simulink model "BD_PAR_AUTO_base_model"  (Simulink 10.3)
settings: Solver=ode1  StartTime=0.0  StopTime=max(cyc_mph(:,1))  FixedStep=1  MaxStep=1  RelTol=1e-3  AbsTol=1e-3
undefined symbols (not defined in the file): acc_dcdc_eff, acc_elec_eff, acc_elec_pwr, acc_mech_eff, acc_mech_pwr, acc_mech_trq, air_cp, amb_tmp, cs_charge_deplete_bool, cs_charge_trq, cs_electric_decel_spd, cs_electric_launch_spd_hi, cs_electric_launch_spd_lo, cs_hi_soc, cs_lo_soc, cs_min_trq_frac, cs_off_trq_frac, cyc_avg_time, cyc_cargo_mass, cyc_elevation_init, cyc_filter_bool, cyc_grade, cyc_mph, enable_sim_stop_distance, enable_sim_stop_max_spd, enable_sim_stop_speed, enable_sim_stop_time, enable_stop, enable_stop_fc, ess_cap_scale, ess_coulombic_eff, ess_init_soc, ess_max_ah_cap, ess_max_volts, ess_min_volts, ess_mod_airflow, ess_mod_cp, ess_mod_init_tmp, ess_module_mass, ess_module_num, ess_on, ess_r_chg, ess_r_dis, ess_res_scale_coef, ess_res_scale_fun, ess_set_tmp, ess_soc, ess_th_calc, ess_th_res_off, ess_th_res_on, ess_tmp, ess_voc, ex_calc, ex_cat_co_frac, ex_cat_ext_cp, ex_cat_ext_emisv, ex_cat_ext_init_tmp, ex_cat_ext_mass, ex_cat_ext_sarea, ex_cat_hc_frac ... (+168)
(part 7 of 15)

== system BD_PAR_AUTO_base_model/energy storage <ess>/ess config/energy storage <ess>/pack Voc, Rint ==
  SOC (prev) : Inport
  req'd battery power (W) : Inport  Port=2
  mod tmp   (C) : Inport  Port=3
  #bty : Constant  Value=ess_module_num
  Product : Product  InputSameDT=on  RndMeth=Zero  SaturateOnIntegerOverflow=on  OutDataTypeStr=Inherit: Same as first input
  Rchg (ohms) : Subsystem  mask(2-D Table Lookup){xindex=ess_tmp, yindex=ess_soc, table=ess_r_chg}
      mask prompts: xindex "X Index"; yindex "Y Index"
      mask help:
      | Two Dimensional Table Lookup
      | The first input corresponds to X Index and the second input corresponds to the Y Index
      mask init:
      | sftab2chk(xindex,yindex,table);
      mask Help: This block returns a linearly interpolated intersection from the table using the X index (which corresponds to the rows of the table) and the Y index (which corresponds to the columns of the table).  Extrapolation is used.
      mask Display: plot(-10,-10,110,110,[90,50,10],[90,40,30],[90,50,10],[50,26,20],[90,50,10],[22,13,10])
  Rdis (ohms) : Subsystem  mask(2-D Table Lookup){xindex=ess_tmp, yindex=ess_soc, table=ess_r_dis}
      mask prompts: xindex "X Index"; yindex "Y Index"
      mask help:
      | Two Dimensional Table Lookup
      | The first input corresponds to X Index and the second input corresponds to the Y Index
      mask init:
      | sftab2chk(xindex,yindex,table);
      mask Help: This block returns a linearly interpolated intersection from the table using the X index (which corresponds to the rows of the table) and the Y index (which corresponds to the columns of the table).  Extrapolation is used.
      mask Display: plot(-10,-10,110,110,[90,50,10],[90,40,30],[90,50,10],[50,26,20],[90,50,10],[22,13,10])
  Switch : Switch
  VOC (V) : Subsystem  mask(2-D Table Lookup){xindex=ess_tmp, yindex=ess_soc, table=ess_voc}
      mask prompts: xindex "X Index"; yindex "Y Index"
      mask help:
      | Two Dimensional Table Lookup
      | The first input corresponds to X Index and the second input corresponds to the Y Index
      mask init:
      | sftab2chk(xindex,yindex,table);
      mask Help: This block returns a linearly interpolated intersection from the table using the X index (which corresponds to the rows of the table) and the Y index (which corresponds to the columns of the table).  Extrapolation is used.
      mask Display: plot(-10,-10,110,110,[90,50,10],[90,40,30],[90,50,10],[50,26,20],[90,50,10],[22,13,10])
  resistance scale fun : Gain  Gain=ess_res_scale_fun(ess_res_scale_coef,ess_module_num,ess_cap_scale)  SaturateOnIntegerOverflow=on  OutDataTypeStr=Inherit: Same as input  ParamDataTypeStr=Inherit: Same as input
  resistance scale fun1 : Gain  Gain=ess_res_scale_fun(ess_res_scale_coef,ess_module_num,ess_cap_scale)  SaturateOnIntegerOverflow=on  OutDataTypeStr=Inherit: Same as input  ParamDataTypeStr=Inherit: Same as input
  pack open- circuit voltage : Outport  InitialOutput=0
  pack resistance : Outport  Port=2  InitialOutput=0
  wires:
  resistance scale fun1/1 -> Switch/3
  Rchg (ohms)/1(table out) -> resistance scale fun1/1
  resistance scale fun/1 -> Switch/1
  Rdis (ohms)/1(table out) -> resistance scale fun/1
  Switch/1 -> pack resistance/1
  #bty/1 -> Product/2
  Product/1 -> pack open- circuit voltage/1
  VOC (V)/1(table out) -> Product/1
  req'd battery power (W)/1 -> Switch/2
  SOC (prev)/1 -> VOC (V)/2(y0), Rdis (ohms)/2(y0), Rchg (ohms)/2(y0)
  mod tmp   (C)/1 -> VOC (V)/1(x0), Rdis (ohms)/1(x0), Rchg (ohms)/1(x0)

== system BD_PAR_AUTO_base_model/energy storage <ess>/ess config/energy storage <ess>/stop sim ==
  SOC : Inport
  Enable : EnablePort
  Const : Constant  Value=.001
  Relational Operator : RelationalOperator  Operator=<  RndMeth=Nearest  InputSameDT=on
  Stop Simulation : Stop
  wires:
  Const/1 -> Relational Operator/2
  SOC/1 -> Relational Operator/1
  Relational Operator/1 -> Stop Simulation/1

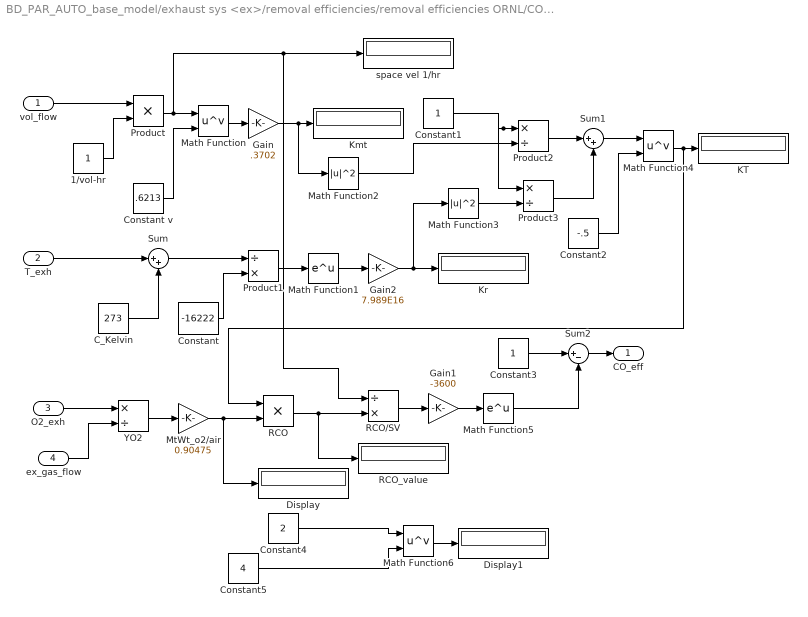
== system BD_PAR_AUTO_base_model/exhaust sys <ex>/removal efficiencies/removal efficiencies ORNL/CO-Conversion ==
  vol_flow : Inport
  T_exh : Inport  Port=2
  O2_exh : Inport  Port=3
  ex_gas_flow : Inport  Port=4
  1/vol-hr : Constant
  C_Kelvin : Constant  Value=273
  Constant : Constant  Value=-16222
  Constant v : Constant  Value=.6213
  Constant1 : Constant
  Constant2 : Constant  Value=-.5
  Constant3 : Constant
  Constant4 : Constant  Value=2
  Constant5 : Constant  Value=4
  Display : Display
  Display1 : Display
  Gain : Gain  Gain=.3702  SaturateOnIntegerOverflow=on
  Gain1 : Gain  Gain=-3600  SaturateOnIntegerOverflow=on
  Gain2 : Gain  Gain=7.989E16  SaturateOnIntegerOverflow=on
  KT : Display
      settings: Format=short_e
  Kmt : Display
      settings: Format=short_e
  Kr : Display
  Math Function : Math  Operator=pow
  Math Function1 : Math
  Math Function2 : Math  Operator=magnitude^2
  Math Function3 : Math  Operator=magnitude^2
  Math Function4 : Math  Operator=pow
  Math Function5 : Math
  Math Function6 : Math  Operator=pow
  MtWt_o2/air : Gain  Gain=0.90475  SaturateOnIntegerOverflow=on
  Product : Product  SaturateOnIntegerOverflow=on
  Product1 : Product  Inputs=/*  SaturateOnIntegerOverflow=on
  Product2 : Product  Inputs=*/  SaturateOnIntegerOverflow=on
  Product3 : Product  Inputs=*/  SaturateOnIntegerOverflow=on
  RCO : Product  SaturateOnIntegerOverflow=on
  RCO/SV : Product  Inputs=/*  SaturateOnIntegerOverflow=on
  RCO_value : Display
  Sum : Sum  Inputs=|++  SaturateOnIntegerOverflow=on
  Sum1 : Sum  Inputs=|++  SaturateOnIntegerOverflow=on
  Sum2 : Sum  Inputs=|+-  SaturateOnIntegerOverflow=on
  YO2 : Product  Inputs=*/  SaturateOnIntegerOverflow=on
  space vel 1/hr : Display
      settings: Format=short_e
  CO_eff : Outport
  wires:
  Math Function6/1 -> Display1/1
  Constant5/1 -> Math Function6/2
  Constant4/1 -> Math Function6/1
  MtWt_o2/air/1 -> Display/1, RCO/2
  YO2/1 -> MtWt_o2/air/1
  RCO/1 -> RCO_value/1, RCO/SV/2
  Sum2/1 -> CO_eff/1
  Math Function5/1 -> Sum2/2
  Constant3/1 -> Sum2/1
  Gain1/1 -> Math Function5/1
  RCO/SV/1 -> Gain1/1
  Math Function4/1 -> RCO/1, KT/1
  ex_gas_flow/1 -> YO2/2
  O2_exh/1 -> YO2/1
  T_exh/1 -> Sum/1
  vol_flow/1 -> Product/1
  Product1/1 -> Math Function1/1
  Constant2/1 -> Math Function4/2
  Sum1/1 -> Math Function4/1
  Product3/1 -> Sum1/2
  Product2/1 -> Sum1/1
  Math Function3/1 -> Product3/2
  Math Function2/1 -> Product2/2
  Constant1/1 -> Product2/1, Product3/1
  Gain2/1 -> Math Function3/1, Kr/1
  Gain/1 -> Math Function2/1, Kmt/1
  Math Function1/1 -> Gain2/1
  Sum/1 -> Product1/1
  Constant/1 -> Product1/2
  C_Kelvin/1 -> Sum/2
  Product/1 -> RCO/SV/1, space vel 1/hr/1, Math Function/1
  Math Function/1 -> Gain/1
  Constant v/1 -> Math Function/2
  1/vol-hr/1 -> Product/2

== system BD_PAR_AUTO_base_model/exhaust sys <ex>/removal efficiencies/removal efficiencies ORNL/HC-Conversion ==
  vol_flow : Inport
  T_exh : Inport  Port=2
  O2_exh : Inport  Port=3
  ex_gas_flow : Inport  Port=4
  1/vol-hr : Constant
  C_Kelvin : Constant  Value=273
  Constant : Constant  Value=-10956
  Constant v : Constant  Value=.6436
  Constant2 : Constant  Value=-.1
  Constant3 : Constant
  Constant4 : Constant  Value=-2171
  Constant5 : Constant  Value=5.818
  Constant6 : Constant  Value=-10
  Gain1 : Gain  Gain=-3600  SaturateOnIntegerOverflow=on
  Gain2 : Gain  Gain=3.731E11  SaturateOnIntegerOverflow=on
  KT : Display
      settings: Format=short_e
  Kmt : Display
      settings: Format=short_e
  Kr : Display
  Math Function{,2..4} (4 alike) : Math  Operator=pow
  Math Function1 : Math
  Math Function5 : Math
  Math Function6 : Math
  MtWt_o2/air : Gain  Gain=0.90475  SaturateOnIntegerOverflow=on
  Product : Product  SaturateOnIntegerOverflow=on
  Product1 : Product  Inputs=/*  SaturateOnIntegerOverflow=on
  Product4 : Product  Inputs=*/  SaturateOnIntegerOverflow=on
  Product5 : Product  Inputs=3  SaturateOnIntegerOverflow=on
  RHC : Product  SaturateOnIntegerOverflow=on
  RHC/SV : Product  Inputs=/*  SaturateOnIntegerOverflow=on
  RHC_value : Display
  Sum : Sum  Inputs=|++  SaturateOnIntegerOverflow=on
  Sum1 : Sum  Inputs=|++  SaturateOnIntegerOverflow=on
  Sum2 : Sum  Inputs=|+-  SaturateOnIntegerOverflow=on
  YO2 : Product  Inputs=*/  SaturateOnIntegerOverflow=on
  space vel 1/hr : Display
      settings: Format=short_e
  HC_eff : Outport
  wires:
  Sum/1 -> Product4/2, Product1/1
  T_exh/1 -> Sum/1
  Math Function3/1 -> Sum1/2
  Math Function2/1 -> Sum1/1
  Constant6/1 -> Math Function3/2, Math Function2/2
  Math Function6/1 -> Product5/3
  Constant5/1 -> Product5/1
  Product4/1 -> Math Function6/1
  Constant4/1 -> Product4/1
  RHC/1 -> RHC_value/1, RHC/SV/2
  MtWt_o2/air/1 -> RHC/2
  YO2/1 -> MtWt_o2/air/1
  Sum2/1 -> HC_eff/1
  Math Function5/1 -> Sum2/2
  Constant3/1 -> Sum2/1
  Gain1/1 -> Math Function5/1
  RHC/SV/1 -> Gain1/1
  Math Function4/1 -> RHC/1, KT/1
  ex_gas_flow/1 -> YO2/2
  O2_exh/1 -> YO2/1
  vol_flow/1 -> Product/1
  Product1/1 -> Math Function1/1
  Constant2/1 -> Math Function4/2
  Sum1/1 -> Math Function4/1
  Gain2/1 -> Math Function3/1, Kr/1
  Product5/1 -> Math Function2/1, Kmt/1
  Math Function1/1 -> Gain2/1
  Constant/1 -> Product1/2
  C_Kelvin/1 -> Sum/2
  Product/1 -> RHC/SV/1, space vel 1/hr/1, Math Function/1
  Math Function/1 -> Product5/2
  Constant v/1 -> Math Function/2
  1/vol-hr/1 -> Product/2

== system BD_PAR_AUTO_base_model/exhaust sys <ex>/removal efficiencies/removal efficiencies ORNL/NOx_Eff ==
  vol_flow : Inport
  Ex_temp : Inport  Port=2
  HC_Inlet : Inport  Port=3
  NOx_Inlet : Inport  Port=4
  1 : Constant
  >eps : Saturate  UpperLimit=inf  LowerLimit=eps
  Gain : Gain  Gain=2.875  SaturateOnIntegerOverflow=on
  Gain1 : Gain  Gain=.01  SaturateOnIntegerOverflow=on
  HNR : Product  Inputs=*/  SaturateOnIntegerOverflow=on
  HNR^.5 : Math  Operator=sqrt
  HNR^2 : Math  Operator=square
  HNR^3 : Product  SaturateOnIntegerOverflow=on
  NOx_conv2 : Display
  SV^.5 : Math  Operator=sqrt
  SV^2 : Math  Operator=square
  SV^3 : Product  SaturateOnIntegerOverflow=on
  Saturation : Saturate  UpperLimit=1.0  LowerLimit=0.0
  Sum : Sum  Inputs=|+++++  SaturateOnIntegerOverflow=on
  Sum1 : Sum  Inputs=|++++  SaturateOnIntegerOverflow=on
  Sum2 : Sum  Inputs=|++++  SaturateOnIntegerOverflow=on
  Sum3 : Sum  Inputs=|+++  SaturateOnIntegerOverflow=on
  TR : Product  Inputs=*/  SaturateOnIntegerOverflow=on
  T^-.5 : Math  Operator=sqrt
  T^-2 : Math  Operator=square
  T^-3 : Product  SaturateOnIntegerOverflow=on
  b0 : Constant  Value=-1.2477959e2
  b1 : Gain  Gain=-6.671239E-4  SaturateOnIntegerOverflow=on
  b10 : Gain  Gain=-1.7874225E1  SaturateOnIntegerOverflow=on
  b11 : Gain  Gain=-2.0607707  SaturateOnIntegerOverflow=on
  b12 : Gain  Gain=1.3883777E-1  SaturateOnIntegerOverflow=on
  b13 : Gain  SaturateOnIntegerOverflow=on
  b2 : Gain  Gain=8.308073E-2  SaturateOnIntegerOverflow=on
  b3 : Gain  Gain=7.9852675E-9  SaturateOnIntegerOverflow=on
  b4 : Gain  Gain=-3.7023358E-14  SaturateOnIntegerOverflow=on
  b5 : Gain  Gain=-5.4929168E4  SaturateOnIntegerOverflow=on
  b6 : Gain  Gain=4.9229015e3  SaturateOnIntegerOverflow=on
  b7 : Gain  Gain=2.959987e6  SaturateOnIntegerOverflow=on
  b8 : Gain  Gain=-1.022441e8  SaturateOnIntegerOverflow=on
  b9 : Gain  Gain=1.3710201E1  SaturateOnIntegerOverflow=on
  NOx_eff : Outport
  wires:
  >eps/1 -> HNR/2
  NOx_Inlet/1 -> >eps/1
  Saturation/1 -> NOx_eff/1, NOx_conv2/1
  Ex_temp/1 -> TR/2
  HC_Inlet/1 -> HNR/1
  b13/1 -> SV^3/1, b1/1, SV^2/1, SV^.5/1
  Gain1/1 -> Saturation/1
  Sum3/1 -> Gain1/1
  Gain/1 -> HNR^2/1, HNR^3/2, b9/1, HNR^.5/1
  HNR/1 -> Gain/1
  Sum/1 -> Sum3/1
  Sum1/1 -> Sum3/2
  Sum2/1 -> Sum3/3
  b12/1 -> Sum2/4
  b11/1 -> Sum2/3
  b10/1 -> Sum2/2
  b9/1 -> Sum2/1
  HNR^.5/1 -> b10/1
  HNR^2/1 -> b11/1, HNR^3/1
  HNR^3/1 -> b12/1
  b8/1 -> Sum1/4
  b7/1 -> Sum1/3
  b6/1 -> Sum1/2
  b5/1 -> Sum1/1
  T^-.5/1 -> b6/1
  T^-2/1 -> b7/1, T^-3/1
  T^-3/1 -> b8/1
  TR/1 -> b5/1, T^-3/2, T^-2/1, T^-.5/1
  1/1 -> TR/1
  b3/1 -> Sum/5
  b4/1 -> Sum/4
  b1/1 -> Sum/3
  b2/1 -> Sum/2
  b0/1 -> Sum/1
  SV^.5/1 -> b2/1
  SV^2/1 -> b3/1, SV^3/2
  SV^3/1 -> b4/1
  vol_flow/1 -> b13/1

== system BD_PAR_AUTO_base_model/fuel converter  <fc>/engine speed estimator/no-lag Reset Integrator/dt ==
  Clock : Clock
  Memory1 : Memory  InitialCondition=-0.1
  Sum1 : Sum  Inputs=+-  InputSameDT=on  SaturateOnIntegerOverflow=on  OutDataTypeStr=Inherit: Same as first input
  out_1 : Outport  InitialOutput=0
  wires:
  Sum1/1 -> out_1/1
  Memory1/1 -> Sum1/2
  Clock/1 -> Memory1/1, Sum1/1

== system BD_PAR_AUTO_base_model/fuel converter  <fc>/engine torque/effect of inertia (Nm)/Block NOTES ==
  note: Torque required to accelerate the engine inertia is taken from the engine
      | acceleration, and is assumed to be no less than zero if the trace was missed
      | at all on the previous time step.
      |
      | The torque required to accelerate the engine's inertia is never assumed to
      | be more than the product of the engine's maximum torque and the engine's
      | contribution to the total vehicle inertia.

== system BD_PAR_AUTO_base_model/fuel converter  <fc>/engine torque/effect of inertia (Nm)/engine inertia as a function of total vehicle inertia (generous approximation) ==
  Product : Product  Inputs=*/  InputSameDT=on  RndMeth=Zero  SaturateOnIntegerOverflow=on  OutDataTypeStr=Inherit: Same as first input
  Sum : Sum  Inputs=++|  InputSameDT=on  SaturateOnIntegerOverflow=on  OutDataTypeStr=Inherit: Same as first input
  engine inertia as a fraction of total vehicle inertia  (generous approximation)--denomenator : Fcn  Expr=fc_inertia*(u*fd_ratio/wh_radius)^2
  engine inertia as a fraction of total vehicle inertia  (generous approximation)--numerator : Fcn  Expr=fc_inertia*(u*fd_ratio/wh_radius)^2
  veh mass calc : Subsystem
  Out1 : Outport
  wires:
  [gear_ratio] -> engine inertia as a fraction of total vehicle inertia  (generous approximation)--numerator/1, engine inertia as a fraction of total vehicle inertia  (generous approximation)--denomenator/1
  veh mass calc/1(Out1) -> Sum/1
  engine inertia as a fraction of total vehicle inertia  (generous approximation)--denomenator/1 -> Sum/2
  engine inertia as a fraction of total vehicle inertia  (generous approximation)--numerator/1 -> Product/1
  Sum/1 -> Product/2
  Product/1 -> Out1/1

== system BD_PAR_AUTO_base_model/fuel converter  <fc>/fuel use and EO emis Configurable Subsystem/fuel use and EO emis/Block NOTES ==
  note: This block determines actual fuel use and engine-out emissions
      | given the fully hot values and the engine coolant temperature.
      | The correlations used here were developed at NREL using
      | FTP data collected under subcontract by JDM & Associates.
      | Note: PM hot/cold relation assumed same as HC

== system BD_PAR_AUTO_base_model/fuel converter  <fc>/fuel use and EO emis Configurable Subsystem/fuel use and EO emis/HOT engine maps  ==
  T (Nm) : Inport
  w (rad/s) : Inport  Port=2
  Enable : EnablePort  StatesWhenEnabling=reset
  Block NOTES : Subsystem
      mask Display: disp('Block\nNOTES')
  CO (g/s) : Subsystem  mask(2-D Table Lookup){xindex=fc_map_spd*fc_spd_scale, yindex=fc_map_trq*fc_trq_scale, table=fc_co_map*fc_spd_scale*fc_trq_scale}
      mask prompts: xindex "X Index"; yindex "Y Index"
      mask help:
      | Two Dimensional Table Lookup
      | The first input corresponds to X Index and the second input corresponds to the Y Index
      mask init:
      | sftab2chk(xindex,yindex,table);
      mask Help: This block returns a linearly interpolated intersection from the table using the X index (which corresponds to the rows of the table) and the Y index (which corresponds to the columns of the table).  Extrapolation is used.
      mask Display: plot(-10,-10,110,110,[90,50,10],[90,40,30],[90,50,10],[50,26,20],[90,50,10],[22,13,10])
  Fcn3 : Fcn  Expr=(u(1)/1000)*ex_gas_cp*(u(2) - amb_tmp)
  HC (g/s) : Subsystem  mask(2-D Table Lookup){xindex=fc_map_spd*fc_spd_scale, yindex=fc_map_trq*fc_trq_scale, table=fc_hc_map*fc_spd_scale*fc_trq_scale}
      mask prompts: xindex "X Index"; yindex "Y Index"
      mask help:
      | Two Dimensional Table Lookup
      | The first input corresponds to X Index and the second input corresponds to the Y Index
      mask init:
      | sftab2chk(xindex,yindex,table);
      mask Help: This block returns a linearly interpolated intersection from the table using the X index (which corresponds to the rows of the table) and the Y index (which corresponds to the columns of the table).  Extrapolation is used.
      mask Display: plot(-10,-10,110,110,[90,50,10],[90,40,30],[90,50,10],[50,26,20],[90,50,10],[22,13,10])
  MF,ex (g/s) : Subsystem  mask(2-D Table Lookup){xindex=fc_map_spd*fc_spd_scale, yindex=fc_map_trq*fc_trq_scale, table=fc_exflow_map*fc_spd_scale*fc_trq_scale}
      mask prompts: xindex "X Index"; yindex "Y Index"
      mask help:
      | Two Dimensional Table Lookup
      | The first input corresponds to X Index and the second input corresponds to the Y Index
      mask init:
      | sftab2chk(xindex,yindex,table);
      mask Help: This block returns a linearly interpolated intersection from the table using the X index (which corresponds to the rows of the table) and the Y index (which corresponds to the columns of the table).  Extrapolation is used.
      mask Display: plot(-10,-10,110,110,[90,50,10],[90,40,30],[90,50,10],[50,26,20],[90,50,10],[22,13,10])
  MinMax : MinMax  Inputs=2  InputSameDT=on  SaturateOnIntegerOverflow=on
  Mux : Mux
  Mux4 : Mux  Inputs=2
  NOx (g/s) : Subsystem  mask(2-D Table Lookup){xindex=fc_map_spd*fc_spd_scale, yindex=fc_map_trq*fc_trq_scale, table=fc_nox_map*fc_spd_scale*fc_trq_scale}
      mask prompts: xindex "X Index"; yindex "Y Index"
      mask help:
      | Two Dimensional Table Lookup
      | The first input corresponds to X Index and the second input corresponds to the Y Index
      mask init:
      | sftab2chk(xindex,yindex,table);
      mask Help: This block returns a linearly interpolated intersection from the table using the X index (which corresponds to the rows of the table) and the Y index (which corresponds to the columns of the table).  Extrapolation is used.
      mask Display: plot(-10,-10,110,110,[90,50,10],[90,40,30],[90,50,10],[50,26,20],[90,50,10],[22,13,10])
  O2 (g/s) : Subsystem  mask(2-D Table Lookup){xindex=fc_map_spd*fc_spd_scale, yindex=fc_map_trq*fc_trq_scale, table=fc_o2_map*fc_spd_scale*fc_trq_scale}
      mask prompts: xindex "X Index"; yindex "Y Index"
      mask help:
      | Two Dimensional Table Lookup
      | The first input corresponds to X Index and the second input corresponds to the Y Index
      mask init:
      | sftab2chk(xindex,yindex,table);
      mask Help: This block returns a linearly interpolated intersection from the table using the X index (which corresponds to the rows of the table) and the Y index (which corresponds to the columns of the table).  Extrapolation is used.
      mask Display: plot(-10,-10,110,110,[90,50,10],[90,40,30],[90,50,10],[50,26,20],[90,50,10],[22,13,10])
  PM (g/s) : Subsystem  mask(2-D Table Lookup){xindex=fc_map_spd*fc_spd_scale, yindex=fc_map_trq*fc_trq_scale, table=fc_pm_map*fc_spd_scale*fc_trq_scale}
      mask prompts: xindex "X Index"; yindex "Y Index"
      mask help:
      | Two Dimensional Table Lookup
      | The first input corresponds to X Index and the second input corresponds to the Y Index
      mask init:
      | sftab2chk(xindex,yindex,table);
      mask Help: This block returns a linearly interpolated intersection from the table using the X index (which corresponds to the rows of the table) and the Y index (which corresponds to the columns of the table).  Extrapolation is used.
      mask Display: plot(-10,-10,110,110,[90,50,10],[90,40,30],[90,50,10],[50,26,20],[90,50,10],[22,13,10])
  Product : Product  InputSameDT=on  RndMeth=Zero  SaturateOnIntegerOverflow=on  OutDataTypeStr=Inherit: Same as first input
  Saturation : Saturate  UpperLimit=max(fc_map_trq*fc_trq_scale)  LowerLimit=min(fc_map_trq*fc_trq_scale)
  Saturation1 : Saturate  UpperLimit=max(fc_map_spd*fc_spd_scale)  LowerLimit=min(fc_map_spd*fc_spd_scale)
  Sum5 : Sum  Inputs=-+  InputSameDT=on  SaturateOnIntegerOverflow=on  OutDataTypeStr=Inherit: Same as first input
  Sum6 : Sum  Inputs=-+  InputSameDT=on  SaturateOnIntegerOverflow=on  OutDataTypeStr=Inherit: Same as first input
  Tex,eo (C) : Subsystem  mask(2-D Table Lookup){xindex=fc_map_spd*fc_spd_scale, yindex=fc_map_trq*fc_trq_scale, table=fc_extmp_map}
      mask prompts: xindex "X Index"; yindex "Y Index"
      mask help:
      | Two Dimensional Table Lookup
      | The first input corresponds to X Index and the second input corresponds to the Y Index
      mask init:
      | sftab2chk(xindex,yindex,table);
      mask Help: This block returns a linearly interpolated intersection from the table using the X index (which corresponds to the rows of the table) and the Y index (which corresponds to the columns of the table).  Extrapolation is used.
      mask Display: plot(-10,-10,110,110,[90,50,10],[90,40,30],[90,50,10],[50,26,20],[90,50,10],[22,13,10])
  fuel (g/s) : Subsystem  mask(2-D Table Lookup){xindex=fc_map_spd*fc_spd_scale, yindex=fc_map_trq*fc_trq_scale, table=fc_fuel_map*fc_spd_scale*fc_trq_scale/fc_eff_scale}
      mask prompts: xindex "X Index"; yindex "Y Index"
      mask help:
      | Two Dimensional Table Lookup
      | The first input corresponds to X Index and the second input corresponds to the Y Index
      mask init:
      | sftab2chk(xindex,yindex,table);
      mask Help: This block returns a linearly interpolated intersection from the table using the X index (which corresponds to the rows of the table) and the Y index (which corresponds to the columns of the table).  Extrapolation is used.
      mask Display: plot(-10,-10,110,110,[90,50,10],[90,40,30],[90,50,10],[50,26,20],[90,50,10],[22,13,10])
  lhv : Gain  Gain=fc_fuel_lhv  SaturateOnIntegerOverflow=on  OutDataTypeStr=Inherit: Same as input  ParamDataTypeStr=Inherit: Same as input
  fc heat (W) : Outport  OutputWhenDisabled=reset  InitialOutput=eps
  HOT fuel use (g/s) : Outport  Port=2  OutputWhenDisabled=reset  InitialOutput=eps
  HOT emis (g/s) : Outport  Port=3  OutputWhenDisabled=reset  InitialOutput=eps
  Ex Gas Flow (g/s) : Outport  Port=4  OutputWhenDisabled=reset  InitialOutput=eps
  Ex Gas Temp (C) : Outport  Port=5  OutputWhenDisabled=reset  InitialOutput=amb_tmp
  O2 exhaust (g/s) : Outport  Port=6  OutputWhenDisabled=reset  InitialOutput=0
  ex heat (W) : Outport  Port=7  OutputWhenDisabled=reset  InitialOutput=eps
  wires:
  O2 (g/s)/1(table out) -> O2 exhaust (g/s)/1
  lhv/1 -> Sum6/2
  fuel (g/s)/1(table out) -> lhv/1, HOT fuel use (g/s)/1
  Product/1 -> Sum6/1
  Sum6/1 -> MinMax/2, Sum5/2
  MinMax/1 -> ex heat (W)/1, Sum5/1
  Fcn3/1 -> MinMax/1
  Sum5/1 -> fc heat (W)/1
  Mux4/1 -> Fcn3/1
  w (rad/s)/1 -> Product/2, Saturation1/1
  T (Nm)/1 -> Product/1, Saturation/1
  Saturation/1 -> HC (g/s)/2(y0), NOx (g/s)/2(y0), PM (g/s)/2(y0), O2 (g/s)/2(y0), fuel (g/s)/2(y0), Tex,eo (C)/2(y0), MF,ex (g/s)/2(y0), CO (g/s)/2(y0)
  Saturation1/1 -> HC (g/s)/1(x0), CO (g/s)/1(x0), PM (g/s)/1(x0), O2 (g/s)/1(x0), fuel (g/s)/1(x0), Tex,eo (C)/1(x0), MF,ex (g/s)/1(x0), NOx (g/s)/1(x0)
  Tex,eo (C)/1(table out) -> Mux4/2, Ex Gas Temp (C)/1
  MF,ex (g/s)/1(table out) -> Mux4/1, Ex Gas Flow (g/s)/1
  Mux/1 -> HOT emis (g/s)/1
  NOx (g/s)/1(table out) -> Mux/3
  CO (g/s)/1(table out) -> Mux/2
  HC (g/s)/1(table out) -> Mux/1
  PM (g/s)/1(table out) -> Mux/4

== system BD_PAR_AUTO_base_model/fuel converter  <fc>/fuel use and EO emis Configurable Subsystem/fuel use and EO emis/fc temp ==
  note: c
  note: i
  note: x
  note: h
  veh spd (m/s) : Inport
  key ON? : Inport  Port=2
  fc ON? : Inport  Port=3
  Qfc (W) : Inport  Port=4
  "1/ " : Gain  Gain=1/(0.2*fc_base_mass*fc_pwr_scale*fc_cp)  SaturateOnIntegerOverflow=on  OutDataTypeStr=Inherit: Same as input  ParamDataTypeStr=Inherit: Same as input
  1/Ci : Gain  Gain=1/(0.8*fc_base_mass*fc_pwr_scale*fc_cp)  SaturateOnIntegerOverflow=on  OutDataTypeStr=Inherit: Same as input  ParamDataTypeStr=Inherit: Same as input
  1/Cx : Gain  Gain=1/(fc_acc_mass*fc_pwr_scale*fc_cp)  SaturateOnIntegerOverflow=on  OutDataTypeStr=Inherit: Same as input  ParamDataTypeStr=Inherit: Same as input
  1/mcp : Gain  Gain=1/(0.1*veh_glider_mass*fc_pwr_scale*fc_h_cp)  SaturateOnIntegerOverflow=on  OutDataTypeStr=Inherit: Same as input  ParamDataTypeStr=Inherit: Same as input
  Block NOTES : Subsystem
      mask Display: disp('Block\nNOTES')
  Memory : Memory  InitialCondition=fc_h_init_tmp
  Mux3 : Mux
  Mux4 : Mux  Inputs=2
  Qc : Sum  InputSameDT=on  SaturateOnIntegerOverflow=on  OutDataTypeStr=Inherit: Same as first input
  Qc1 : Sum  Inputs=--+  InputSameDT=on  SaturateOnIntegerOverflow=on  OutDataTypeStr=Inherit: Same as first input
  Tcm : Integrator  InitialCondition=fc_c_init_tmp
  Tcx : Integrator  InitialCondition=fc_x_init_tmp
  Tcx1 : Integrator  InitialCondition=fc_i_init_tmp
  Tm : Integrator  InitialCondition=fc_h_init_tmp
  fc coolant : Subsystem  TreatAsAtomicUnit=on
  fc mass heat flow : Subsystem
  old fc coolant  temp. (C) : Subsystem
  Tfc_old  (C) : Outport  InitialOutput=0
  Qfc r,h : Outport  Port=2  InitialOutput=0
  Tfc  (C) : Outport  Port=3  InitialOutput=0
  tag scope: fc_hood_temp=global
  wires:
  Memory/1 -> [fc_hood_temp]
  fc ON?/1 -> old fc coolant  temp. (C)/1(fc on?)
  veh spd (m/s)/1 -> fc mass heat flow/1(veh spd), old fc coolant  temp. (C)/2(veh spd)
  old fc coolant  temp. (C)/1(fc coolant  temp (C)) -> Tfc_old  (C)/1
  Mux3/1 -> Tfc  (C)/1, fc mass heat flow/2(fc_temp)
  fc mass heat flow/4(Qfc_h) -> 1/mcp/1
  1/mcp/1 -> Tm/1
  Tm/1 -> Memory/1, Mux3/4
  Tcx/1 -> Mux3/3
  key ON?/1 -> fc coolant/Enable
  fc mass heat flow/3(Qfc_x) -> 1/Cx/1
  1/Cx/1 -> Tcx/1
  Mux4/1 -> Qfc r,h/1
  Tcx1/1 -> Mux3/2, fc coolant/1(Tcl)
  fc coolant/1(Qfc_rad) -> Mux4/1, Qc1/1
  fc coolant/2(Qfc_htr) -> Mux4/2, Qc1/2
  fc mass heat flow/2(Qfc_i) -> fc coolant/2("Qfc_i "), Qc1/3
  Tcm/1 -> Mux3/1
  1/Ci/1 -> Tcx1/1
  Qc1/1 -> 1/Ci/1
  fc mass heat flow/1(Qfc_c) -> Qc/2
  Qfc (W)/1 -> Qc/1
  "1/ "/1 -> Tcm/1
  Qc/1 -> "1/ "/1

== system BD_PAR_AUTO_base_model/fuel converter  <fc>/fuel use and EO emis Configurable Subsystem/fuel use and EO emis/fc temp correct ==
  Coolant T (C) : Inport
  HOT fuel use (g/s) : Inport  Port=2
  HOT emis (g/s) : Inport  Port=3
  T (Nm) : Inport  Port=4
  w (rad/s) : Inport  Port=5
  Enable : EnablePort  StatesWhenEnabling=reset
  =1: use map based =0: use constant equation based : Constant  Value=fc_cold
  Switch : Switch  Threshold=eps
  Switch1 : Switch  Threshold=eps
  fc temp correct Constant Correction Factors (Equation Based) : Subsystem  TreatAsAtomicUnit=on
  fc temp correct Variable Correction Factors (Map Based) : Subsystem  TreatAsAtomicUnit=on
  fc_cold=0 : Logic  Operator=NOT
  fuel use (g/s) : Outport  OutputWhenDisabled=reset  InitialOutput=0
  EO emis (g/s) : Outport  Port=2  OutputWhenDisabled=reset  InitialOutput=0
  wires:
  w (rad/s)/1 -> fc temp correct Variable Correction Factors (Map Based)/5(w (rad/s))
  T (Nm)/1 -> fc temp correct Variable Correction Factors (Map Based)/4(T (Nm))
  Switch1/1 -> EO emis (g/s)/1
  Switch/1 -> fuel use (g/s)/1
  fc temp correct Variable Correction Factors (Map Based)/2(EO emis (g/s)) -> Switch1/3
  fc temp correct Constant Correction Factors (Equation Based)/2(EO emis (g/s)) -> Switch1/1
  fc temp correct Variable Correction Factors (Map Based)/1(fuel use (g/s)) -> Switch/3
  fc_cold=0/1 -> Switch1/2, Switch/2, fc temp correct Constant Correction Factors (Equation Based)/Enable
  fc temp correct Constant Correction Factors (Equation Based)/1(fuel use (g/s)) -> Switch/1
  HOT emis (g/s)/1 -> fc temp correct Variable Correction Factors (Map Based)/3(HOT emis (g/s)), fc temp correct Constant Correction Factors (Equation Based)/3(HOT emis (g/s))
  HOT fuel use (g/s)/1 -> fc temp correct Variable Correction Factors (Map Based)/2(HOT fuel use (g/s)), fc temp correct Constant Correction Factors (Equation Based)/2(HOT fuel use (g/s))
  Coolant T (C)/1 -> fc temp correct Variable Correction Factors (Map Based)/1(Coolant T (C)), fc temp correct Constant Correction Factors (Equation Based)/1(Coolant T (C))
  =1: use map based =0: use constant equation based/1 -> fc temp correct Variable Correction Factors (Map Based)/Enable, fc_cold=0/1

== system BD_PAR_AUTO_base_model/gearbox <gb>/Pout/Pin, neglecting inertia/make division bombproof/Block NOTES ==
  note: this block added 10 July 2001 by mpo:
      | originally a -eps was added to the denominator by default.
      | However, cases were ecountered where Tin-Tineratia was equal to -eps causing
      | the denominator to be zero. This added checking is more rhobust

== system BD_PAR_AUTO_base_model/hydraulic torque converter for  parallel hybrid <htc>/T, shifting/T_max/Block NOTES ==
  note: Notes: engine_on flag causes algebric loop. Is it necessary?
      | Doesn't seem to be. Disabled 10/31/00:tm

== system BD_PAR_AUTO_base_model/mechanical accessory loads <acc>/Mechanical Accessory Loads v2 <acc>/Accessory SDO/mechanical power logging ==
  In1 : Inport
  Gain : Gain  Gain=acc_mech_eff  SaturateOnIntegerOverflow=on  OutDataTypeStr=Inherit: Same as input  ParamDataTypeStr=Inherit: Same as input
  To Workspace6 : ToWorkspace  VariableName=acc_mech_pwr_in_a  SampleTime=-1
  To Workspace8 : ToWorkspace  VariableName=acc_mech_pwr_out_a  SampleTime=-1
  wires:
  Gain/1 -> To Workspace8/1
  In1/1 -> Gain/1, To Workspace6/1

== system BD_PAR_AUTO_base_model/mechanical accessory loads <acc>/Mechanical Accessory Loads v2 <acc>/backward model/mechanical accessories (Nm) ==
  w_APU : Inport
  Mechanical Accessories: Const Mech Var Elect : Subsystem
      mask Display: image(imread('bdi_acc_pic_cs.bmp'))
  T_acc : Outport
  P_mech_acc : Outport  Port=2
  probes : Outport  Port=3
  wires:
  w_APU/1 -> Mechanical Accessories: Const Mech Var Elect/1(w_APU)
  Mechanical Accessories: Const Mech Var Elect/1(T_acc) -> T_acc/1
  Mechanical Accessories: Const Mech Var Elect/2(P_mech_acc) -> P_mech_acc/1
  Mechanical Accessories: Const Mech Var Elect/3(probes) -> probes/1

== system BD_PAR_AUTO_base_model/motor/ controller <mc> par/effect of inertia (Nm)/motor inertia as a function of total vehicle inertia (generous approximation)/veh mass calc ==
  Constant : Constant  Value=veh_mass
  Sum : Sum  Inputs=|++  SaturateOnIntegerOverflow=on
  Out1 : Outport
  wires:
  Sum/1 -> Out1/1
  Constant/1 -> Sum/2
  [veh_cargo_mass] -> Sum/1

== system BD_PAR_AUTO_base_model/vehicle <veh>/record achieved force outputs/force req'd to accelerate (N)1/current veh mass ==
  Constant3 : Constant  Value=veh_mass
  Sum1 : Sum  Inputs=|++  SaturateOnIntegerOverflow=on
  Out1 : Outport
  wires:
  Constant3/1 -> Sum1/1
  [veh_cargo_mass] -> Sum1/2
  Sum1/1 -> Out1/1

== system BD_PAR_AUTO_base_model/vehicle <veh>/record achieved force outputs/force req'd to ascend (N)1/current veh mass ==
  Constant3 : Constant  Value=veh_mass
  Sum1 : Sum  Inputs=|++  SaturateOnIntegerOverflow=on
  Out1 : Outport
  wires:
  Constant3/1 -> Sum1/1
  [veh_cargo_mass] -> Sum1/2
  Sum1/1 -> Out1/1

== system BD_PAR_AUTO_base_model/vehicle <veh>/record achieved force outputs/rolling resistance force/force req'd to overcome rolling resistance (N) ==
  average vehicle speed over time step (m/s) : Inport
  Constant : Constant  Value=wh_1st_rrc
  Constant1 : Constant  Value=0
  Constant2 : Constant  Value=veh_gravity
  Gain1 : Gain  Gain=wh_2nd_rrc  SaturateOnIntegerOverflow=on
  Product : Product  Inputs=4  SaturateOnIntegerOverflow=on
  Sum : Sum  SaturateOnIntegerOverflow=on
  Switch : Switch  Threshold=eps
  Trig Fn2 : Trigonometry  Operator=atan
  Trig Fn3 : Trigonometry  Operator=cos
  current veh mass : Subsystem
  Fr (N) : Outport  InitialOutput=0
  wires:
  Constant/1 -> Sum/1
  Gain1/1 -> Sum/2
  Switch/1 -> Fr (N)/1
  average vehicle speed over time step (m/s)/1 -> Gain1/1, Switch/2
  Constant1/1 -> Switch/3
  Sum/1 -> Product/2
  Constant2/1 -> Product/1
  Product/1 -> Switch/1
  Trig Fn3/1 -> Product/3
  current veh mass/1(Out1) -> Product/4
  [grade] -> Trig Fn2/1
  Trig Fn2/1 -> Trig Fn3/1

== system BD_PAR_AUTO_base_model/vehicle <veh>/rolling resistance force/force req'd to overcome rolling resistance (N)/current veh mass ==
  Constant3 : Constant  Value=veh_mass
  Sum1 : Sum  Inputs=|++  SaturateOnIntegerOverflow=on
  Out1 : Outport
  wires:
  Constant3/1 -> Sum1/1
  [veh_cargo_mass] -> Sum1/2
  Sum1/1 -> Out1/1

== system BD_PAR_AUTO_base_model/vehicle <veh>/vehicle speed/vehicle speed (m/s)/Block NOTES ==
  note: Given the tractive force available, this block uses straightforward vehicle
      | dynamics equations to determine the achievable speed.
  note: The actual vehicle speed at the end of the time step is taken as
      | the LESSER of the speed computed from the actual force and the speed
      | computed from the actual drivetrain speed if the required acceleration
      |  is greater than -1 m/s^2.  Otherwise, the GREATER of the two values is used.
      | Thus the worse acceleration rate is allowed if the vehicle is accelerating,
      | and the worse deceleration rate is allowed if the vehicle is decelerating.
      |
      | In no case will the computed speed fall below zero.

== system BD_PAR_AUTO_base_model/vehicle <veh>/vehicle speed/vehicle speed (m/s)/b ==
  dt : Inport
  angle of elevation : Inport  Port=2
  vehicle moving? : Inport  Port=3
  Constant9 : Constant  Value=veh_gravity*wh_2nd_rrc
  Gain : Gain  Gain=2  SaturateOnIntegerOverflow=on
  Product10 : Product  Inputs=4  SaturateOnIntegerOverflow=on
  Product6 : Product  Inputs=*/  SaturateOnIntegerOverflow=on
  Sum : Sum  SaturateOnIntegerOverflow=on
  Trig Fn7 : Trigonometry  Operator=cos
  current veh mass : Subsystem
  current veh mass1 : Subsystem
  b : Outport
  wires:
  Gain/1 -> Product6/1
  Product6/1 -> Sum/1
  Trig Fn7/1 -> Product10/2
  Constant9/1 -> Product10/1
  Product10/1 -> Sum/2
  Sum/1 -> b/1
  dt/1 -> Product6/2
  angle of elevation/1 -> Trig Fn7/1
  vehicle moving?/1 -> Product10/3
  current veh mass/1(Out1) -> Gain/1
  current veh mass1/1(Out1) -> Product10/4

== system BD_PAR_AUTO_base_model/vehicle <veh>/vehicle speed/vehicle speed (m/s)/c ==
  note: note: the constant
      | veh_mass used in this block
  dt : Inport
  v_prev : Inport  Port=2
  Ftract : Inport  Port=3
  angle of elevation : Inport  Port=4
  vehicle moving? : Inport  Port=5
  Constant12 : Constant  Value=wh_1st_rrc
  Constant13 : Constant  Value=veh_gravity
  Gain : Gain  Gain=2  SaturateOnIntegerOverflow=on
  Product7 : Product  Inputs=*/*  SaturateOnIntegerOverflow=on
  Product8 : Product  Inputs=3  SaturateOnIntegerOverflow=on
  Product9 : Product  Inputs=3  SaturateOnIntegerOverflow=on
  Sum : Sum  Inputs=--+  SaturateOnIntegerOverflow=on
  Sum6 : Sum  SaturateOnIntegerOverflow=on
  Trig Fn : Trigonometry  Operator=cos
  Trig Fn2 : Trigonometry
  current veh mass : Subsystem
  current veh mass1 : Subsystem
  prevent imaginary #s : Saturate  UpperLimit=inf  LowerLimit=-70*veh_mass
  c : Outport
  wires:
  v_prev/1 -> Product7/3
  Product7/1 -> Sum/1
  prevent imaginary #s/1 -> Sum/2
  Ftract/1 -> prevent imaginary #s/1
  Constant12/1 -> Product9/1
  Trig Fn/1 -> Product9/2
  Product9/1 -> Sum6/1
  angle of elevation/1 -> Trig Fn/1, Trig Fn2/1
  Trig Fn2/1 -> Sum6/2
  vehicle moving?/1 -> Product9/3
  Sum6/1 -> Product8/1
  Constant13/1 -> Product8/2
  Product8/1 -> Sum/3
  Sum/1 -> c/1
  dt/1 -> Product7/2
  Gain/1 -> Product7/1
  current veh mass1/1(Out1) -> Gain/1
  current veh mass/1(Out1) -> Product8/3

== system BD_PAR_AUTO_base_model/vehicle <veh>/vehicle speed/vehicle speed (m/s)/current veh mass ==
  Constant3 : Constant  Value=veh_mass
  Sum1 : Sum  Inputs=|++  SaturateOnIntegerOverflow=on
  Out1 : Outport
  wires:
  Constant3/1 -> Sum1/1
  [veh_cargo_mass] -> Sum1/2
  Sum1/1 -> Out1/1

== system BD_PAR_AUTO_base_model/<vc> par auto/config traction control/traction control 2 axle/apply tire traction limit to req'd speed (m/s)/Block NOTES ==
  note: Front-wheel drive is assumed, and weight transfer due to acceleration is included in the calculation of maximum tractive force.
  note: The above equations are derived by solving F_maxaccel=mass*a_max for the maximum or minimum speed at the end of the time step,
      | given that F_maxaccel depends on the weight borne by the front tires which in turn depends on the vehicle's acceleration rate.
  note: This block limits the requested speed by the maximum and minimum attainable given the maximum traction of the tires.
      | That is, acceleration and braking maneuvers are limited to the point of imminent skidding.

== system BD_PAR_AUTO_base_model/<vc> par auto/config traction control/traction control 2 axle/apply tire traction limit to req'd speed (m/s)/current veh mass (kg) ==
  Constant12 : Constant  Value=veh_mass
  Sum8 : Sum  Inputs=|++  InputSameDT=on  SaturateOnIntegerOverflow=on  OutDataTypeStr=Inherit: Same as first input
  Out1 : Outport
  wires:
  Constant12/1 -> Sum8/2
  [veh_cargo_mass] -> Sum8/1
  Sum8/1 -> Out1/1

== system BD_PAR_AUTO_base_model/<vc> par auto/config traction control/traction control 2 axle/apply tire traction limit to req'd speed (m/s)/current veh mass (kg)1 ==
  Constant12 : Constant  Value=veh_mass
  Sum8 : Sum  Inputs=|++  InputSameDT=on  SaturateOnIntegerOverflow=on  OutDataTypeStr=Inherit: Same as first input
  Out1 : Outport
  wires:
  Constant12/1 -> Sum8/2
  [veh_cargo_mass] -> Sum8/1
  Sum8/1 -> Out1/1

== system BD_PAR_AUTO_base_model/<vc> par auto/config traction control/traction control 2 axle/apply tire traction limit to req'd speed (m/s)/current veh mass (kg)10 ==
  Constant12 : Constant  Value=veh_mass
  Sum8 : Sum  Inputs=|++  InputSameDT=on  SaturateOnIntegerOverflow=on  OutDataTypeStr=Inherit: Same as first input
  Out1 : Outport
  wires:
  Constant12/1 -> Sum8/2
  [veh_cargo_mass] -> Sum8/1
  Sum8/1 -> Out1/1

== system BD_PAR_AUTO_base_model/<vc> par auto/config traction control/traction control 2 axle/apply tire traction limit to req'd speed (m/s)/current veh mass (kg)2 ==
  Constant12 : Constant  Value=veh_mass
  Sum8 : Sum  Inputs=|++  InputSameDT=on  SaturateOnIntegerOverflow=on  OutDataTypeStr=Inherit: Same as first input
  Out1 : Outport
  wires:
  Constant12/1 -> Sum8/2
  [veh_cargo_mass] -> Sum8/1
  Sum8/1 -> Out1/1

== system BD_PAR_AUTO_base_model/<vc> par auto/config traction control/traction control 2 axle/apply tire traction limit to req'd speed (m/s)/current veh mass (kg)3 ==
  Constant12 : Constant  Value=veh_mass
  Sum8 : Sum  Inputs=|++  InputSameDT=on  SaturateOnIntegerOverflow=on  OutDataTypeStr=Inherit: Same as first input
  Out1 : Outport
  wires:
  Constant12/1 -> Sum8/2
  [veh_cargo_mass] -> Sum8/1
  Sum8/1 -> Out1/1

== system BD_PAR_AUTO_base_model/<vc> par auto/config traction control/traction control 2 axle/apply tire traction limit to req'd speed (m/s)/current veh mass (kg)4 ==
  Constant12 : Constant  Value=veh_mass
  Sum8 : Sum  Inputs=|++  InputSameDT=on  SaturateOnIntegerOverflow=on  OutDataTypeStr=Inherit: Same as first input
  Out1 : Outport
  wires:
  Constant12/1 -> Sum8/2
  [veh_cargo_mass] -> Sum8/1
  Sum8/1 -> Out1/1

== system BD_PAR_AUTO_base_model/<vc> par auto/config traction control/traction control 2 axle/apply tire traction limit to req'd speed (m/s)/current veh mass (kg)5 ==
  Constant12 : Constant  Value=veh_mass
  Sum8 : Sum  Inputs=|++  InputSameDT=on  SaturateOnIntegerOverflow=on  OutDataTypeStr=Inherit: Same as first input
  Out1 : Outport
  wires:
  Constant12/1 -> Sum8/2
  [veh_cargo_mass] -> Sum8/1
  Sum8/1 -> Out1/1

== system BD_PAR_AUTO_base_model/<vc> par auto/config traction control/traction control 2 axle/apply tire traction limit to req'd speed (m/s)/current veh mass (kg)6 ==
  Constant12 : Constant  Value=veh_mass
  Sum8 : Sum  Inputs=|++  InputSameDT=on  SaturateOnIntegerOverflow=on  OutDataTypeStr=Inherit: Same as first input
  Out1 : Outport
  wires:
  Constant12/1 -> Sum8/2
  [veh_cargo_mass] -> Sum8/1
  Sum8/1 -> Out1/1

== system BD_PAR_AUTO_base_model/<vc> par auto/config traction control/traction control 2 axle/apply tire traction limit to req'd speed (m/s)/current veh mass (kg)7 ==
  Constant12 : Constant  Value=veh_mass
  Sum8 : Sum  Inputs=|++  InputSameDT=on  SaturateOnIntegerOverflow=on  OutDataTypeStr=Inherit: Same as first input
  Out1 : Outport
  wires:
  Constant12/1 -> Sum8/2
  [veh_cargo_mass] -> Sum8/1
  Sum8/1 -> Out1/1

== system BD_PAR_AUTO_base_model/<vc> par auto/config traction control/traction control 2 axle/apply tire traction limit to req'd speed (m/s)/current veh mass (kg)8 ==
  Constant12 : Constant  Value=veh_mass
  Sum8 : Sum  Inputs=|++  InputSameDT=on  SaturateOnIntegerOverflow=on  OutDataTypeStr=Inherit: Same as first input
  Out1 : Outport
  wires:
  Constant12/1 -> Sum8/2
  [veh_cargo_mass] -> Sum8/1
  Sum8/1 -> Out1/1

== system BD_PAR_AUTO_base_model/<vc> par auto/config traction control/traction control 2 axle/apply tire traction limit to req'd speed (m/s)/max speed at END of time step given tire traction limit (m/s) ==
  in_1 : Inport
  in_2 : Inport  Port=2
  Fcn : Fcn  Expr=1/u
  Product : Product  InputSameDT=on  RndMeth=Zero  SaturateOnIntegerOverflow=on  OutDataTypeStr=Inherit: Same as first input
  out_1 : Outport  InitialOutput=0
  wires:
  in_2/1 -> Fcn/1
  Product/1 -> out_1/1
  Fcn/1 -> Product/2
  in_1/1 -> Product/1

== system BD_PAR_AUTO_base_model/<vc> par auto/config traction control/traction control 2 axle/apply tire traction limit to req'd speed (m/s)/min speed at END of time step given tire traction limit (m/s) ==
  in_1 : Inport
  in_2 : Inport  Port=2
  Fcn : Fcn  Expr=1/u
  Product : Product  InputSameDT=on  RndMeth=Zero  SaturateOnIntegerOverflow=on  OutDataTypeStr=Inherit: Same as first input
  out_1 : Outport  InitialOutput=0
  wires:
  in_1/1 -> Product/1
  Fcn/1 -> Product/2
  Product/1 -> out_1/1
  in_2/1 -> Fcn/1

== system BD_PAR_AUTO_base_model/<vc> par auto/config traction control/traction control 2 axle/apply tire traction limit to req'd speed (m/s)/rear slip terms ==
  initial speed : Inport
  1/dt : Inport  Port=2
  sin(theta) : Inport  Port=3
  Constant12 : Constant  Value=max(wh_slip_force_coeff)*(-1*veh_cg_height)/veh_wheelbase
  Constant8 : Constant  Value=veh_gravity
  Product13 : Product  Inputs=3  InputSameDT=on  RndMeth=Zero  SaturateOnIntegerOverflow=on  OutDataTypeStr=Inherit: Same as first input
  Product14 : Product  Inputs=4  InputSameDT=on  RndMeth=Zero  SaturateOnIntegerOverflow=on  OutDataTypeStr=Inherit: Same as first input
  current  veh mass (kg) : Subsystem
  Out1 : Outport
  Out2 : Outport  Port=2
  wires:
  Constant12/1 -> Product14/1, Product13/1
  Constant8/1 -> Product13/2
  current  veh mass (kg)/1(Out1) -> Product14/4
  initial speed/1 -> Product14/2
  Product14/1 -> Out1/1
  1/dt/1 -> Product14/3
  Product13/1 -> Out2/1
  sin(theta)/1 -> Product13/3

== system BD_PAR_AUTO_base_model/<vc> par auto/config traction control/traction control 2 axle/enforce max.  front axle tractive force  due to slip (N)/Block NOTES ==
  note: No more force will be requested of the drivetrain than can be transmitted by the front tires.
      | This transmittable force is computed taking into account the slip characteristics of the tires
      | and the variable, acceleration-dependent weight borne by the front axle.

== system BD_PAR_AUTO_base_model/<vc> par auto/config traction control/traction control 2 axle/enforce max.  front axle tractive force  due to slip (N)/front ==
  In1 : Inport
  In2 : Inport  Port=2
  Clock : Clock
  Constant : Constant  Value=veh_cg_height/veh_wheelbase
  Constant1 : Constant  Value=veh_gravity*veh_front_wt_frac
  Gain1 : Gain  Gain=2  SaturateOnIntegerOverflow=on  OutDataTypeStr=Inherit: Same as input  ParamDataTypeStr=Inherit: Same as input
  Gain2 : Gain  Gain=veh_gravity  SaturateOnIntegerOverflow=on  OutDataTypeStr=Inherit: Same as input  ParamDataTypeStr=Inherit: Same as input
  Memory1 : Memory  InitialCondition=-0.1
  Product : Product  Inputs=*/  InputSameDT=on  RndMeth=Zero  SaturateOnIntegerOverflow=on  OutDataTypeStr=Inherit: Same as first input
  Product1 : Product  Inputs=3  InputSameDT=on  RndMeth=Zero  SaturateOnIntegerOverflow=on  OutDataTypeStr=Inherit: Same as first input
  Product3 : Product  Inputs=3  InputSameDT=on  RndMeth=Zero  SaturateOnIntegerOverflow=on  OutDataTypeStr=Inherit: Same as first input
  Sum : Sum  Inputs=+-  InputSameDT=on  SaturateOnIntegerOverflow=on  OutDataTypeStr=Inherit: Same as first input
  Sum1 : Sum  Inputs=+-  InputSameDT=on  SaturateOnIntegerOverflow=on  OutDataTypeStr=Inherit: Same as first input
  Sum2 : Sum  InputSameDT=on  SaturateOnIntegerOverflow=on  OutDataTypeStr=Inherit: Same as first input
  Trig Fn : Trigonometry  Operator=atan
  Trig Fn1 : Trigonometry
  Trig Fn2 : Trigonometry  Operator=cos
  current veh mass (kg) : Subsystem
  weight on front axle (N)1 : Sum  Inputs=-+  InputSameDT=on  SaturateOnIntegerOverflow=on  OutDataTypeStr=Inherit: Same as first input
  Out1 : Outport
  wires:
  Product1/1 -> weight on front axle (N)1/1
  Constant/1 -> Product1/1
  Sum/1 -> Product/1
  Clock/1 -> Sum1/1, Memory1/1
  Memory1/1 -> Sum1/2
  Sum1/1 -> Product/2
  Product/1 -> Gain1/1
  Gain1/1 -> Sum2/1
  Sum2/1 -> Product1/2
  [grade] -> Trig Fn/1
  Trig Fn1/1 -> Gain2/1
  Gain2/1 -> Sum2/2
  Trig Fn/1 -> Trig Fn1/1, Trig Fn2/1
  Product3/1 -> weight on front axle (N)1/2
  Constant1/1 -> Product3/3
  Trig Fn2/1 -> Product3/2
  current veh mass (kg)/1(Out1) -> Product1/3, Product3/1
  In1/1 -> Sum/1
  In2/1 -> Sum/2
  weight on front axle (N)1/1 -> Out1/1

== system BD_PAR_AUTO_base_model/<vc> par auto/config traction control/traction control 2 axle/enforce max.  front axle tractive force  due to slip (N)/rear ==
  In1 : Inport
  In2 : Inport  Port=2
  Clock : Clock
  Constant : Constant  Value=(-1*veh_cg_height)/veh_wheelbase
  Constant1 : Constant  Value=veh_gravity*(1-veh_front_wt_frac)
  Gain1 : Gain  Gain=2  SaturateOnIntegerOverflow=on  OutDataTypeStr=Inherit: Same as input  ParamDataTypeStr=Inherit: Same as input
  Gain2 : Gain  Gain=veh_gravity  SaturateOnIntegerOverflow=on  OutDataTypeStr=Inherit: Same as input  ParamDataTypeStr=Inherit: Same as input
  Memory1 : Memory  InitialCondition=-0.1
  Product : Product  Inputs=*/  InputSameDT=on  RndMeth=Zero  SaturateOnIntegerOverflow=on  OutDataTypeStr=Inherit: Same as first input
  Product1 : Product  Inputs=3  InputSameDT=on  RndMeth=Zero  SaturateOnIntegerOverflow=on  OutDataTypeStr=Inherit: Same as first input
  Product3 : Product  Inputs=3  InputSameDT=on  RndMeth=Zero  SaturateOnIntegerOverflow=on  OutDataTypeStr=Inherit: Same as first input
  Sum : Sum  Inputs=+-  InputSameDT=on  SaturateOnIntegerOverflow=on  OutDataTypeStr=Inherit: Same as first input
  Sum1 : Sum  Inputs=+-  InputSameDT=on  SaturateOnIntegerOverflow=on  OutDataTypeStr=Inherit: Same as first input
  Sum2 : Sum  InputSameDT=on  SaturateOnIntegerOverflow=on  OutDataTypeStr=Inherit: Same as first input
  Trig Fn : Trigonometry  Operator=atan
  Trig Fn1 : Trigonometry
  Trig Fn2 : Trigonometry  Operator=cos
  current veh mass (kg) : Subsystem
  weight on rear axle (N) : Sum  Inputs=-+  InputSameDT=on  SaturateOnIntegerOverflow=on  OutDataTypeStr=Inherit: Same as first input
  Out1 : Outport
  wires:
  Product1/1 -> weight on rear axle (N)/1
  Constant/1 -> Product1/1
  Sum/1 -> Product/1
  Clock/1 -> Sum1/1, Memory1/1
  Memory1/1 -> Sum1/2
  Sum1/1 -> Product/2
  Product/1 -> Gain1/1
  Gain1/1 -> Sum2/1
  Sum2/1 -> Product1/2
  [grade] -> Trig Fn/1
  Trig Fn1/1 -> Gain2/1
  Gain2/1 -> Sum2/2
  Trig Fn/1 -> Trig Fn1/1, Trig Fn2/1
  Product3/1 -> weight on rear axle (N)/2
  Constant1/1 -> Product3/3
  Trig Fn2/1 -> Product3/2
  current veh mass (kg)/1(Out1) -> Product1/3, Product3/1
  In1/1 -> Sum/1
  In2/1 -> Sum/2
  weight on rear axle (N)/1 -> Out1/1

== system BD_PAR_AUTO_base_model/<vc> par auto/gearbox control for use w/ AT/Speed Dependent Shifting/shifting/time since last shift ==
  in_1 : Inport
  just shifted : Subsystem
      mask Display: disp('just\nshifted')
  timer : Subsystem
      mask Display: disp('timer')
  out_1 : Outport  InitialOutput=0
  wires:
  timer/1(time) -> out_1/1
  just shifted/1(out_1) -> timer/1(trigger)
  in_1/1 -> just shifted/1(in_1)

== system BD_PAR_AUTO_base_model/<vc> par auto/gearbox control for use w/ AT/Speed Dependent Shifting/shifting1/time since last shift ==
  in_1 : Inport
  just shifted : Subsystem
      mask Display: disp('just\nshifted')
  timer : Subsystem
      mask Display: disp('timer')
  out_1 : Outport  InitialOutput=0
  wires:
  timer/1(time) -> out_1/1
  just shifted/1(out_1) -> timer/1(trigger)
  in_1/1 -> just shifted/1(in_1)
